simulink model "ali_ozkan1"  (Simulink 8.4)
settings: Solver=ode23t  StartTime=0.0  StopTime=0.1  RelTol=1e-3
libraries: powerlib x10, powerlib_meascontrol x4
settings Model: Creator=asus1  LastModifiedBy=asus1
settings DataIOCC: SignalLoggingSaveFormat=Dataset
settings OptimizationCC: ExpressionDepthLimit=128
settings DebuggingCC: UnderspecifiedInitializationDetection=Simplified  MergeDetectMultiDrivingBlocksExec=error  FcnCallInpInsideContextMsg=EnableAllAsError  StateNameClashWarn=none
settings GRTTargetCC: CombineOutputUpdateFcns=on  GRTInterface=off

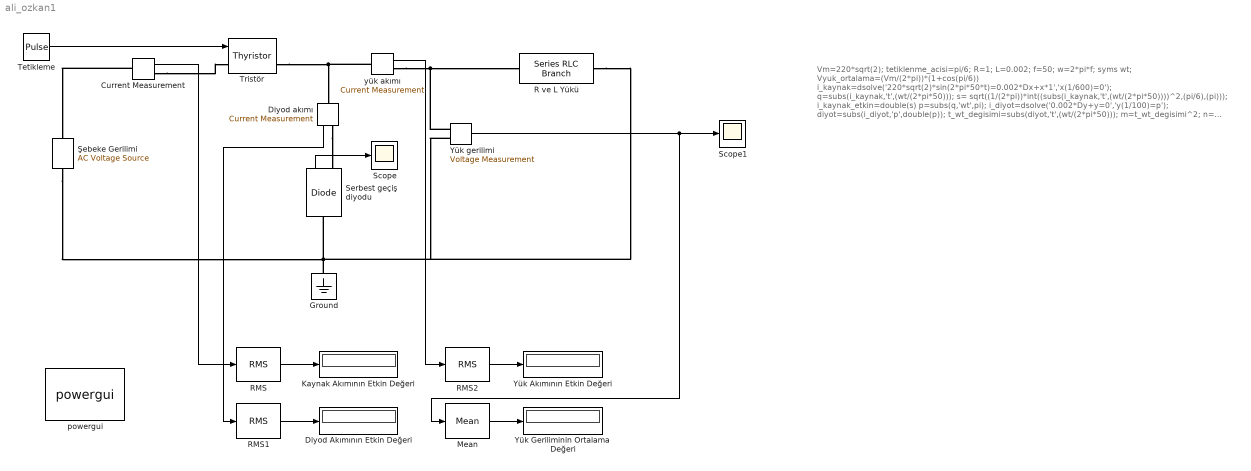
== system ali_ozkan1 ==
  note: Vm=220*sqrt(2);
      | tetiklenme_acisi=pi/6;
      | R=1;
      | L=0.002;
      | f=50;
      | w=2*pi*f;
      | syms wt;
      | Vyuk_ortalama=(Vm/(2*pi))*(1+cos(pi/6))
      | i_kaynak=dsolve('220*sqrt(2)*sin(2*pi*50*t)=0.002*Dx+x*1','x(1/600)=0');
      | q=subs(i_kaynak,'t',(wt/(2*pi*50)));
      | s= sqrt((1/(2*pi))*int((subs(i_kaynak,'t',(wt/(2*pi*50))))^2,(pi/6),(pi)));
      | i_kaynak_etkin=double(s)
      | p=subs(q,'wt',pi);
      | i_diyot=dsolve('0.002*Dy+y=0','y(1/100)=p');
      | diyot=subs(i_diyot,'p',double(p));
      | t_wt_degisimi=subs(diyot,'t',(wt/(2*pi*50)));
      | m=t_wt_degisimi^2;
      | n= sqrt((1/(2*pi))*int(m,pi,(2*pi)));
      | diyot_akimi_etkin=double(n)
      | yuk_akimi_etkin=sqrt(((i_kaynak_etkin)^2)+((diyot_akimi_etkin)^2))
  Current Measurement : powerlib/Measurements/Current Measurement  PhasorSimulation=off  OutputType=Complex  PSBequivalent=0
  Diyod Akımının Etkin Değeri : Display
  Diyod akımı : powerlib/Measurements/Current Measurement  PhasorSimulation=off  OutputType=Complex  PSBequivalent=0
  Ground : powerlib/Elements/Ground  LConnTagsString=a
  Kaynak Akımının Etkin Değeri : Display
  Mean : powerlib_meascontrol/Measurements/Mean  Freq=50  Vinit=0  Ts=0
  R ve L Yükü : powerlib/Elements/Series RLC Branch  LConnTagsString=__new0  RConnTagsString=__new0  BranchType=RL  Resistance=1  Inductance=2e-3  SetiL0=off  InitialCurrent=0  Capacitance=1e-6  Setx0=off  InitialVoltage=0  Measurements=None
  RMS : powerlib_meascontrol/Measurements/RMS  TrueRMS=on  Freq=50  RMSInit=120  Ts=0
  RMS1 : powerlib_meascontrol/Measurements/RMS  TrueRMS=on  Freq=50  RMSInit=120  Ts=0
  RMS2 : powerlib_meascontrol/Measurements/RMS  TrueRMS=on  Freq=50  RMSInit=120  Ts=0
  Scope : Scope
  Scope1 : Scope
  Serbest geçiş diyodu : powerlib/Power Electronics/Diode  Ron=0.00000001  Lon=0  Vf=0  IC=0  UseSnubber=off  Rs=5000  Cs=250e-9  Measurements=on
  "Tetikleme " : DiscretePulseGenerator  PulseType=Time based  Period=0.02  PulseWidth=50  PhaseDelay=0.0016666
  "Tristör " : powerlib/Power Electronics/Thyristor  Ron=0.0000001  Lon=0  Vf=0  IC=0  Rs=5000  Cs=250e-9  Measurements=on
  Yük Akımının Etkin Değeri : Display
  Yük Geriliminin Ortalama Değeri : Display
  "Yük gerilimi " : powerlib/Measurements/Voltage Measurement  PhasorSimulation=off  OutputType=Complex  PSBequivalent=0
  powergui : powerlib/powergui  Priority=1  SimulationMode=Discrete  SolverType=Tustin  SampleTime=50e-7  frequency=60  SPID=off  DisableSnubberDevices=off  DisableRonSwitches=off  DisableVfSwitches=off  SwTol=0  DisplayEquations=off  Interpol=off  methode=off  Ts=100  frequencyindice=50  Pbase=100e6  ErrMax=1e-4  Iterations=50  UnitsV=kV  UnitsW=MW  FunctionMessages=off  echomessages=off  HookPort=off  EnableUseOfTLC=off  x0status=blocks  RestoreLinks=warning  ResistiveCurrentMeasurement=off  Frange=[0:2:500]  Ylog=off  Xlog=on  ShowGrid=off  save=off  variable=ZData  structure=0  ZoomFFT=off  StartTime=0.0  cycles=1  DisplayStyle=1  fundamental=60  FreqAxis=off  MaxFrequency=1000  frequencyindicesteady=1  RmsSteady=1  display=off
  yük akımı : powerlib/Measurements/Current Measurement  PhasorSimulation=off  OutputType=Complex  PSBequivalent=0
  Şebeke Gerilimi : powerlib/Electrical Sources/AC Voltage Source  Amplitude=310  Phase=0  Frequency=50  SampleTime=0  Measurements=None
  wires:
  "Tetikleme "/1 -> "Tristör "/1
  Current Measurement/1 -> RMS/1
  Diyod akımı/1 -> RMS1/1
  RMS/1 -> Kaynak Akımının Etkin Değeri/1
  RMS1/1 -> Diyod Akımının Etkin Değeri/1
  yük akımı/1 -> RMS2/1
  RMS2/1 -> Yük Akımının Etkin Değeri/1
  Mean/1 -> Yük Geriliminin Ortalama Değeri/1
  Serbest geçiş diyodu/1 -> Scope/1
  "Yük gerilimi "/1 -> Mean/1, Scope1/1
  connections:
  Current Measurement/RConn1 -- "Tristör "/LConn1
  Current Measurement/LConn1 -- Şebeke Gerilimi/RConn1
  "Tristör "/RConn1 -- yük akımı/LConn1 -- Diyod akımı/LConn1
  Diyod akımı/RConn1 -- Serbest geçiş diyodu/RConn1
  Şebeke Gerilimi/LConn1 -- Ground/LConn1 -- R ve L Yükü/RConn1 -- "Yük gerilimi "/LConn2 -- Serbest geçiş diyodu/LConn1
  yük akımı/RConn1 -- R ve L Yükü/LConn1 -- "Yük gerilimi "/LConn1
